simulink model "untitled"  (R2018a)
settings: Solver=FixedStepAuto  StartTime=0.0  StopTime=10.0  RelTol=1e-3
settings Model: Creator=Yulou  LastModifiedBy=Yulou
settings OptimizationCC: DefaultParameterBehavior=Inlined  UseDivisionForNetSlopeComputation=on  UseFloatMulNetSlope=on  InlineInvariantSignals=on  PassReuseOutputArgsAs=Individual arguments  ZeroExternalMemoryAtStartup=off  ZeroInternalMemoryAtStartup=off  NoFixptDivByZeroProtection=on  EfficientFloat2IntCast=on  LifeSpan=1  OptimizeBlockOrder=speed  DifferentSizesBufferReuse=on
settings DebuggingCC: ParameterTunabilityLossMsg=error
settings HardwareCC: ProdLongLongMode=on
settings SFSimCC: MATLABDynamicMemAlloc=off
settings RTWCC: SystemTargetFile=ert.tlc  TemplateMakefile=ert_default_tmf  GenerateReport=on  IncludeHyperlinkInReport=on  LaunchReport=on  TargetLang=C++  GenerateTraceInfo=on  GenerateTraceReport=on  GenerateTraceReportSl=on  GenerateTraceReportSf=on  GenerateTraceReportEml=on
settings CodeAppCC: ForceParamTrailComments=on  IgnoreCustomStorageClasses=off  OperatorAnnotations=on  SimulinkDataObjDesc=on  SFDataObjDesc=on  CustomSymbolStrGlobalVar=rt$N$M  CustomSymbolStrType=$N$M  CustomSymbolStrFcn=$N$M$F  CustomSymbolStrMacro=$N$M  InsertBlockDesc=on
settings ERTTargetCC: TargetLangStandard=C++03 (ISO)  GenerateSampleERTMain=on  IncludeMdlTerminateFcn=off  CombineSignalStateStructs=on  SupportAbsoluteTime=off  MultiInstanceERTCode=on  CodeInterfacePackaging=C++ class  SupportComplex=off  SupportNonInlinedSFcns=on  InlinedParameterPlacement=NonHierarchical  RootIOFormat=Structure reference  ERTCustomFileTemplate=example_file_process.tlc  ERTFilePackagingFormat=CompactWithDataFile

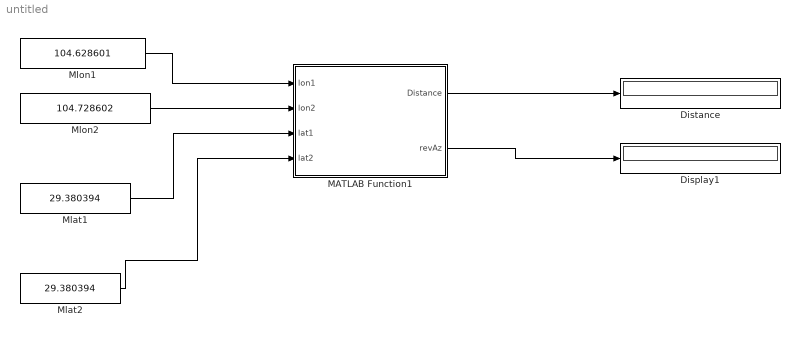
== system untitled ==
  Display1 : Display
  Distance : Display
  MATLAB Function1 : MATLAB Function  TreatAsAtomicUnit=on
  Mlat1 : Constant  Value=29.380394  OutDataTypeStr=double
  "Mlat2 " : Constant  Value=29.380394  OutDataTypeStr=double
  Mlon1 : Constant  Value=104.628601  OutDataTypeStr=double
  Mlon2 : Constant  Value=104.728602  OutDataTypeStr=double
  wires:
  Mlon1/1 -> MATLAB Function1/1(lon1)
  Mlon2/1 -> MATLAB Function1/2(lon2)
  Mlat1/1 -> MATLAB Function1/3(lat1)
  "Mlat2 "/1 -> MATLAB Function1/4(lat2)
  MATLAB Function1/1(Distance) -> Distance/1
  MATLAB Function1/2(revAz) -> Display1/1

== matlab function untitled/MATLAB Function1 ==
  data: lon1 input; Distance output; lon2 input; lat1 input; lat2 input; revAz output
function [Distance, revAz] = fcn(lon1, lon2, lat1, lat2)
   
R=6371.004;
radLat1 = deg2rad(lat1);
radLat2 = deg2rad(lat2);
radLon1 = deg2rad(lon1);
radLon2 = deg2rad(lon2);
a = radLat1 - radLat2;
b = radLon1 - radLon2;
h=haversin(a)+cos(radLat1)*cos(radLat2)*haversin(b);
Distance = 2 * R * asin(sqrt(h));

lon1 = deg2rad(lon1) ; lat1 = deg2rad(lat1);  %p1	
lon2 = deg2rad(lon2); lat2 = deg2rad(lat2);   %p2

f = 1 /  298.257223563;
a= 6378137.0;	
b= 6356752.314245;

L = lon2 - lon1;
tanU1 = (1-f)*tan(lat1); cosU1 = 1 / sqrt((1 + tanU1*tanU1));sinU1 = tanU1 * cosU1;
tanU2 = (1-f)*tan(lat2); cosU2 = 1 / sqrt((1 + tanU2*tanU2));sinU2 = tanU2 * cosU2;
lambda = L;
lambda_ = 0;
iterationLimit = 100;
cosSq_alpha = 0;
sin_delta = 0;
cos2_deltaM = 0;
cos_delta = 0;
delta = 0;
sinlambda = 0;
coslambda = 0;
while (abs(lambda - lambda_) > 1e-12 && iterationLimit>0)
        iterationLimit = iterationLimit -1;
        sinlambda = sin(lambda);
        coslambda = cos(lambda);
        sinSq_delta = (cosU2*sinlambda) * (cosU2*sinlambda) + (cosU1*sinU2-sinU1*cosU2* coslambda) * (cosU1*sinU2-sinU1*cosU2* coslambda);
        sin_delta = sqrt(sinSq_delta);
        if sin_delta==0 
            revAz = 0;
               return 
        end
        cos_delta = sinU1*sinU2 + cosU1*cosU2*coslambda;
        delta = atan2(sin_delta, cos_delta);
        sin_alpha = cosU1 * cosU2 * sinlambda / sin_delta;
        cosSq_alpha = 1 - sin_alpha*sin_alpha;
        cos2_deltaM = cos_delta - 2*sinU1*sinU2/cosSq_alpha;
        C = f/16*cosSq_alpha*(4+f*(4-3*cosSq_alpha));
        lambda_ = lambda;
        lambda = L + (1-C) * f * sin_alpha * (delta + C*sin_delta*(cos2_deltaM+C*cos_delta*(-1+2*cos2_deltaM*cos2_deltaM)));
end
uSq = cosSq_alpha * (a*a - b*b) / (b*b);
A = 1 + uSq/16384*(4096+uSq*(-768+uSq*(320-175*uSq)));
B = uSq/1024 * (256+uSq*(-128+uSq*(74-47*uSq)));
delta_delta = B*sin_delta*(cos2_deltaM+B/4*(cos_delta*(-1+2*cos2_deltaM*cos2_deltaM)-B/6*cos2_deltaM*(-3+4*sin_delta*sin_delta)*(-3+4*cos2_deltaM*cos2_deltaM)));
s = b*A*(delta-delta_delta);
fwdAz = atan2(cosU2*sinlambda,  cosU1*sinU2-sinU1*cosU2*coslambda); %初始方位角
revAz = atan2(cosU1*sinlambda, -sinU1*cosU2+cosU1*sinU2*coslambda); %最终方位角
end



function y = deg2rad(x)
y = x*pi/180;
end

function z = haversin(x)
z=sin(x/2)^2;
end
